simulink model "model_2_2"  (R2021b)
settings: Solver=FixedStepAuto  StartTime=0.0  StopTime=0.5  FixedStep=0.0000005  RelTol=1e-3
settings Model: Creator=den  LastModifiedBy=den

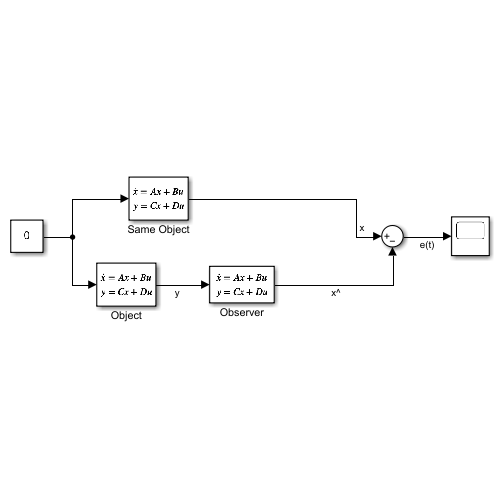
[thumbnail: Simulink's stored preview of the top-level diagram]
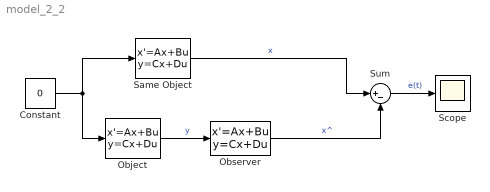
== system model_2_2 ==
  Constant : Constant  Value=0
  Object : StateSpace  A=[0 5 0 0; -5 0 0 0; 0 0 0 1; 0 0 -1 0]  B=[0; 0; 0; 0]  C=[0 9 1 0]  D=0  InitialCondition=[1;1;1;1]
  Observer : StateSpace  A=[0 -1070555/24 -1070675/216 0; -5 1002725/8 1002725/72 0; 0 -9070101/8 -1007789/8 1; 0 -23970333/8 -7990135/24 0]  B=[1070675/216; -1002725/72; 1007789/8; 7990111/24]  C=[1 0 0 0; 0 1 0 0; 0 0 1 0; 0 0 0 1]  D=[0;0;0;0]  InitialCondition=[2;0;0;-1]
  Same Object : StateSpace  A=[0 5 0 0; -5 0 0 0; 0 0 0 1; 0 0 -1 0]  B=[0; 0; 0; 0]  C=[1 0 0 0; 0 1 0 0; 0 0 1 0; 0 0 0 1]  D=[0;0;0;0]  InitialCondition=[1;1;1;1]
  Scope : Scope
  Sum : Sum  Inputs=|+-
  wires:
  Object/1 -> Observer/1  "y"
  Observer/1 -> Sum/2  "x^"
  Constant/1 -> Same Object/1, Object/1
  Same Object/1 -> Sum/1  "x"
  Sum/1 -> Scope/1  "e(t)"
